simulink model "ObjectTrackerHDL_ew"  (R2024b)
settings: Solver=VariableStepAuto  StartTime=0.0  StopTime=0.2  RelTol=1e-3  EnableMultiTasking=on
PreLoadFcn:
  | % Blank input
  | img = zeros(480,640);
  | 
  | % Initialize ROI and its center
  | ROI = [175 270 127 127];
  | center = [ROI(2)+(ROI(4)+1)/2 ROI(1)+(ROI(3)+1)/2];
  | 
  | % Template Size
  | templateSize = 128;
  | tSize = templateSize;
  | 
  | % Learning rate
  | eta = 0.075;
  | 
  | % Number of training images
  | trainCount = 2;
  | 
  | % Gaussian Variance
  | sig = 2;
  | 
  | % Generate a Gaussian centered on the first frame
  | iSize = size(img);
  | [x,y] = ndgrid(1:iSize(1), 1:iSize(2));
  | gauss = exp(-((x-center(1)).^2 + (y-center(2)).^2)./(2*sig));
  | gauss = mat2gray(gauss);
  | 
  | % Generate the first template
  | img = imcrop(img, ROI);
  | gauss = imcrop(gauss, ROI);
  | 
  | % Generate the preprocess windowing function
  | [w1,w2] = meshgrid(window(@hann,tSize),window(@hann,tSize));
  | win = w1.*w2;
  | 
  | % Blank initial coefficients
  | G = zeros(tSize,tSize);
  | Ai = zeros(tSize,tSize);
  | Bi = zeros(tSize,tSize);
  | Hi = zeros(tSize,tSize);
  | 
  | numRows = tSize;
  | numCols = tSize;
InitFcn:
  | % Read the first frame
  | vidFReader = VideoReader(get_param('ObjectTrackerHDL/Input','inputFilename'));
  | img = read(vidFReader,1);
  | if (size(img,3) == 3)
  |     img = rgb2gray(img);
  | end
  | img = double(img);
  | 
  | % Initialize Object Center
  | objectCenter = str2num(get_param('ObjectTrackerHDL/ObjectTrackerHDL','objectCenter'));
  | 
  | % Template Size
  | templateSize = str2num(get_param('ObjectTrackerHDL/ObjectTrackerHDL','templateSize'));
  | originROI = objectCenter-templateSize/2;
  | tSize = templateSize;
  | 
  | % Initialize ROI and its center
  | ROI = [originROI tSize-1 tSize-1];
  | center = [ROI(2)+(ROI(4)+1)/2 ROI(1)+(ROI(3)+1)/2];
  | 
  | % Learning rate
  | eta = 0.075;
  | 
  | % Number of training images
  | trainCount = 128;
  | 
  | % Gaussian Variance
  | sig = 2;
  | 
  | % Generate a Gaussian centered on the first frame
  | iSize = size(img);
  | [x,y] = ndgrid(1:iSize(1), 1:iSize(2));
  | gauss = exp(-((x-center(1)).^2 + (y-center(2)).^2)./(2*sig));
  | gauss = mat2gray(gauss);
  | 
  | % Generate the first template
  | img = imcrop(img, ROI);
  | gauss = imcrop(gauss, ROI);
  | 
  | % Generate the preprocess windowing function
  | [w1,w2] = meshgrid(window(@hann,tSize),window(@hann,tSize));
  | win = w1.*w2;
  | 
  | % Preprocessing the first template
  | hgamma = vision.GammaCorrector(2.0,'Correction','De-gamma');
  | img = hgamma(uint8(img));
  | img = double(img);
  | mean1 = mean(img(:));
  | std1 = std(img(:));
  | img = (img-mean1)/std1;
  | fii = img.*win;
  | 
  | % Convert to frequency domain and calculate initial coefficients
  | G = fft2(gauss);
  | Ai = (G.*conj(fft2(fii)));
  | Bi = real((fft2(fii).*conj(fft2(fii))));
  | 
  | rng('default');
  | % Initial training procedure
  | for i = 1:trainCount
  |     rotateRand = 20.*rand - 10;
  |     resizeRand = 0.2.*rand + 0.9;
  |     img = imresize(imresize(imrotate(img, rotateRand), resizeRand), [tSize tSize]);
  |     img = hgamma(uint8(img));
  |     img = double(img);
  |     img = (img-mean(img(:)))/std(img(:));
  |     fii = img.*win;
  |     Ai = Ai + (G.*conj(fft2(fii)));
  |     Bi = Bi + real((fft2(fii).*conj(fft2(fii))));
  | end
  | 
  | % Initial Filter coefficients
  | Ai = eta.*Ai;
  | Bi = eta.*Bi;
  | Hi = Ai./Bi;
  | 
  | % FFT Parameters
  | numRows = tSize;
  | numCols = tSize;
model workspace (MAT data in the model file):
  mwTaskManagerKernelLatency = 0
undefined symbols (not defined in the file): a, b, c, Rec, SDTV
libraries: hdlsllib x61, simulink x17, visionhdlutilities x8, visionstatistics x6, dsphdlxfrm2 x6, visionconversions x4, visiontransforms x3, visionhdlio x2, visionhdlconversions x2, visionhdlstatistics x2, visionanalysis x2, visionsinks x1
(part 1 of 3)
settings Model: SimulationMode=accelerator  Creator=The MathWorks, Inc.  LastModifiedBy=samet
settings SolverCC: PositivePriorityOrder=on
settings OptimizationCC: BlockReduction=off  ConditionallyExecuteInputs=off  DefaultParameterBehavior=Inlined  EnhancedBackFolding=on  PassReuseOutputArgsAs=Individual arguments  ZeroExternalMemoryAtStartup=off  ZeroInternalMemoryAtStartup=off  MaxStackSize=64  OptimizeBlockOrder=speed  DifferentSizesBufferReuse=on  OptimizationCustomize=off  EfficientTunableParamExpr=on
settings DebuggingCC: AlgebraicLoopMsg=error  ParameterPrecisionLossMsg=none  ParameterTunabilityLossMsg=error  FixptConstOverflowMsg=warning  SubsystemReferenceDiagnosticForUnitTest=warning
settings HardwareCC: ProdBitPerPointer=32  ProdBitPerSizeT=32  ProdBitPerPtrDiffT=32  ProdLargestAtomicFloat=None  ProdIntDivRoundTo=Undefined  ProdEndianess=Unspecified  ProdWordSize=32  ProdHWDeviceType=ASIC/FPGA->ASIC/FPGA  TargetBitPerPointer=64  TargetBitPerSizeT=64  TargetBitPerPtrDiffT=64  TargetLongLongMode=on  TargetIntDivRoundTo=Zero  TargetEndianess=LittleEndian  TargetWordSize=64  TargetHWDeviceType=Custom Processor->MATLAB Host Computer  ProdEqTarget=off  HardwareBoardFeatureSet=SoCBlockset
settings ModelReferenceCC: ModelReferenceNumInstancesAllowed=Single
settings RTWCC: Description=Embedded Coder  SystemTargetFile=ert.tlc  TemplateMakefile=ert_default_tmf  Toolchain=Linaro AArch64 Linux v6.3.1  GPUComputeCapability=3.5
settings CodeAppCC: ForceParamTrailComments=on  IgnoreCustomStorageClasses=off  OperatorAnnotations=on  SimulinkDataObjDesc=on  SFDataObjDesc=on  InsertBlockDesc=on
settings ERTTargetCC: InlinedParameterPlacement=Hierarchical  ERTCustomFileTemplate=example_file_process.tlc  DynamicArrayContainerType=coder::array

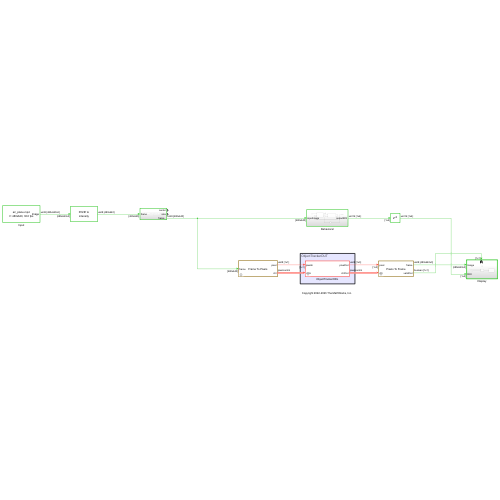
[thumbnail: Simulink's stored preview of the top-level diagram]
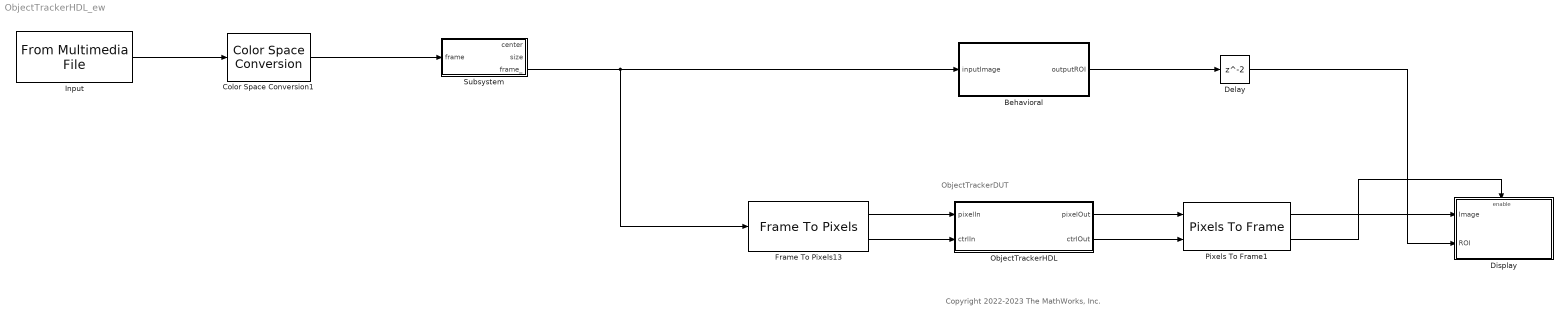
== system ObjectTrackerHDL_ew ==
  note: Copyright 2022-2023 The MathWorks, Inc.
  note: ObjectTrackerDUT
  Behavioral : Subsystem
  Color Space Conversion1 : visionconversions/Color Space  Conversion  conversion=Obsolete  conversionActive=R'G'B' to intensity  wp_str=D65  rec=Rec. 601 (SDTV)  sys=1125/60/2:1  imagePorts=One multidimensional signal
  Delay : Delay
  Display : Subsystem
  Frame To Pixels13 : visionhdlio/Frame To Pixels  NumComponents=1  NumPixels=1  VideoFormat=480p  ActivePixelsPerLine=640  ActiveVideoLines=480  TotalPixelsPerLine=800  TotalVideoLines=525  StartingActiveLine=36  FrontPorch=16  SampleTime=0  VideoFormatCache=480p  ActivePixelsPerLineCache=903  ActiveVideoLinesCache=718  TotalPixelsPerLineCache=950  TotalVideoLinesCache=750  StartingActiveLineCache=6  FrontPorchCache=5
  Input : dspvision/From Multimedia File  inputFilename=C:\Users\samet\OneDrive\Documents\MATLAB\Examples\R2024b\supportfiles\visionhdl\LTIR_dataset\air_plane.mp4  readRange=[1 Inf]  loop=on  numPlays=1  outputStreams=Video only  videoDataType=uint8  audioDataType=int16  inheritSampleTime=on  userDefinedSampleTime=1  noAudioOutput=off  isIntensityVideo=off  fourcc=RGB  colorVideoFormat=One multidimensional signal  outputEOF=off  dataOrg=Column-major  audioFrameSize=1024  computeAudioFrameSize=off  outSamplingMode=Sample based
      settings: LibrarySourceBlock=visionsources/From Multimedia File
  ObjectTrackerHDL : Subsystem  mask{objectCenter=[220 180], templateSize=128, imageSize=iSize}
      mask prompts: objectCenter "Object Center"; templateSize "Template Size"; imageSize "Image Size"
      mask init:
      | % Varsayılan edgeImage matrisi
      |     if evalin('base', 'exist(''edgeImage'', ''var'')') == 0
      |         defaultEdgeImage = false(480, 640); % Varsayılan boş edgeImage matrisi
      |         assignin('base', 'edgeImage', defaultEdgeImage);
      |         fprintf('edgeImage initialized to default zero matrix.\n');
      |     end
      | 
      |     % Retrieve edgeImage from the base workspace
      |     edgeImage = evalin('base', 'edgeImage');
      | 
      |     % Call calculateROI to compute objectCenter and templateSize
      |     try
      |         [objectCenter, templateSize] = calculateROI(edgeImage);
      |     catch ME
      |         error('Error in calculateROI: %s', ME.message);
      |     end
      | 
      |     % Assign computed values to the mask parameters
      |     assignin('base', 'objectCenter', objectCenter);
      |     assignin('base', 'templateSize', templateSize);
      | 
      |     % Debugging information
      |     fprintf('Initialization Complete:\n');
      |     fprintf('Object Center: [%f, %f]\n', objectCenter(1), objectCenter(2));
      |     fprintf('Template Size: %d\n', templateSize);
      mask TypeOptions templateSize: 16 | 32 | 64 | 128 | 256
  Pixels To Frame1 : visionhdlio/Pixels To Frame  NumComponents=3  NumPixels=1  VideoFormat=480p  ActivePixelsPerLine=640  ActiveVideoLines=480  TotalPixelsPerLine=800  TotalVideoLines=525  VideoFormatCache=480p  ActivePixelsPerLineCache=903  ActiveVideoLinesCache=718  TotalPixelsPerLineCache=950  TotalVideoLinesCache=750
  Subsystem : Subsystem
  wires:
  Frame To Pixels13/1 -> ObjectTrackerHDL/1(pixelIn)
  ObjectTrackerHDL/1(pixelOut) -> Pixels To Frame1/1
  ObjectTrackerHDL/2(ctrlOut) -> Pixels To Frame1/2
  Pixels To Frame1/2 -> Display/Enable
  Behavioral/1(outputROI) -> Delay/1
  Delay/1 -> Display/2(ROI)
  Input/1 -> Color Space Conversion1/1
  Frame To Pixels13/2 -> ObjectTrackerHDL/2(ctrlIn)
  Pixels To Frame1/1 -> Display/1(Image)
  Color Space Conversion1/1 -> Subsystem/1(frame)
  Subsystem/3(frame_) -> Frame To Pixels13/1, Behavioral/1(inputImage)

== system ObjectTrackerHDL_ew/Behavioral ==
  inputImage : Inport
  Preprocess : Subsystem
  Terminator : Terminator
  Track : Subsystem
  Transpose : Math  Operator=transpose
  outputROI : Outport
  wires:
  Preprocess/1(outputTemplate) -> Terminator/1
  Transpose/1 -> outputROI/1
  Preprocess/4(outputROI) -> Transpose/1
  inputImage/1 -> Preprocess/1(inputImage)
  Preprocess/2(prevTemplate) -> Track/1(prevTemplate)
  Preprocess/3(currTemplate) -> Track/2(currTemplate)
  Track/1(prevROI) -> Preprocess/2(prevROI)
  Track/2(currROI) -> Preprocess/3(currROI)

== system ObjectTrackerHDL_ew/Display ==
  Image : Inport
  ROI : Inport  Port=2
  Enable : EnablePort
  Display : visionsinks/To Video Display  windowSizeMode=Normal  openAtMdlStart=on  fullScreen=off  videoWindowX=536805376  videoWindowY=536805376  saveWindowSize=off  videoWindowWidth=1654  videoWindowHeight=1181  inputColorFormat=RGB  inputType=Obsolete  imagePorts=One multidimensional signal  OutputDevice=On-screen video monitor  dataOrg=Column-major  isWindowOpen=off
  VideoOverlay : MATLAB Function  TreatAsAtomicUnit=on
  wires:
  Image/1 -> VideoOverlay/1(img)
  VideoOverlay/1(y) -> Display/1
  ROI/1 -> VideoOverlay/2(ROI)

== system ObjectTrackerHDL_ew/ObjectTrackerHDL ==
  note: 2-D Correlation filter tracking HDL Subsystem
  pixelIn : Inport
  ctrlIn : Inport  Port=2
  Overlay : Subsystem
      settings: PortSchema="{\"entries\":[{\"content\":{\"sides\":[{\"content\":{\"connectorIds\":[\"In1\",\"In2\"]},\"type\":\"ConnectorPlacement.EquallySpacedRectSide\",\"uuid\":\"4b8534fb-eb59-4390-9dd3-f879eee42828\"},{\"content\":{\"connectorIds\":[\"Out1\",\"Out2\",\"Out3\"],\"side\":\"RIGHT\"},\"type\":\"ConnectorPlacement.EquallySpacedRectSide\",\"uuid\":\"fb136db1-f133-4b6e-b626-4dade9ce09b9\"},{\"content\":{\"connectorIds\":[\"In3\"],\"side\":\"TOP\"},\"type\":\"ConnectorPlacement.EquallySpacedRectSide\",\"uuid\":\"99d2356e-62e6-4658-9ddf-d950fdf75b9a\"}]},\"type\":\"ConnectorPlacement.EquallySpacedConnector\",\"uuid\":\"47760993-437f-4ecc-9b42-136ef2d923e2\"}],\"packageUris\":[\"http://schema.mathworks.com/mf0/Connector/R2020b\"],\"version\":\"1.0\"}"
  Preprocess : Subsystem
      settings: PortSchema="{\"entries\":[{\"content\":{\"sides\":[{\"content\":{\"connectorIds\":[\"In1\",\"In2\",\"In3\",\"In4\"]},\"type\":\"ConnectorPlacement.EquallySpacedRectSide\",\"uuid\":\"9cec2fe1-69b9-4dab-94c8-faa7de2288f4\"},{\"content\":{\"connectorIds\":[\"Out1\",\"Out2\",\"Out3\",\"Out4\"],\"side\":\"RIGHT\"},\"type\":\"ConnectorPlacement.EquallySpacedRectSide\",\"uuid\":\"e3a596ea-31b4-4396-a8e6-8b94a53ae325\"},{\"content\":{\"connectorIds\":[\"Out5\"],\"side\":\"TOP\"},\"type\":\"ConnectorPlacement.EquallySpacedRectSide\",\"uuid\":\"e24a773b-b8a7-44fa-b0cf-f932f975dd7c\"},{\"content\":{\"side\":\"BOTTOM\"},\"type\":\"ConnectorPlacement.EquallySpacedRectSide\",\"uuid\":\"5ab59a8a-723b-4ab7-825a-3368d576d645\"}]},\"type\":\"ConnectorPlacement.EquallySpacedConnector\",\"uuid\":\"d74f8764-7932-4caf-a531-fe5bd7d99976\"}],\"packageUris\":[\"http://schema.mathworks.com/mf0/Connector/R2020b\"],\"version\":\"1.0\"}"
  Terminator : Terminator
  Track : Subsystem
      settings: PortSchema="{\"entries\":[{\"content\":{\"sides\":[{\"content\":{\"connectorIds\":[\"In1\",\"In2\",\"In3\",\"In4\"]},\"type\":\"ConnectorPlacement.EquallySpacedRectSide\",\"uuid\":\"1d66b792-d543-473d-8440-e34f5801daf7\"},{\"content\":{\"connectorIds\":[\"Out1\",\"Out2\",\"In5\"],\"side\":\"RIGHT\"},\"type\":\"ConnectorPlacement.EquallySpacedRectSide\",\"uuid\":\"0e22f8bb-e063-4450-b36d-cf632a4b5b95\"},{\"content\":{\"side\":\"TOP\"},\"type\":\"ConnectorPlacement.EquallySpacedRectSide\",\"uuid\":\"c0411b5e-6970-47cf-84b0-714a2a15381e\"},{\"content\":{\"side\":\"BOTTOM\"},\"type\":\"ConnectorPlacement.EquallySpacedRectSide\",\"uuid\":\"e852d354-5e9d-40fe-bda7-81286cac12c5\"}]},\"type\":\"ConnectorPlacement.EquallySpacedConnector\",\"uuid\":\"8d3eada4-8f0a-418d-a426-b3492f84d556\"}],\"packageUris\":[\"http://schema.mathworks.com/mf0/Connector/R2020b\"],\"version\":\"1.0\"}"
  pixelOut : Outport
  ctrlOut : Outport  Port=2
  wires:
  ctrlIn/1 -> Overlay/2(ctrlIn), Track/5(frameCtrl), Preprocess/2(ctrlIn)
  pixelIn/1 -> Overlay/1(pixelIn), Preprocess/1(pixelIn)
  Preprocess/1(prevPixelOut) -> Track/1(prevPixelIn)
  Preprocess/2(prevCtrlOut) -> Track/2(prevCtrlIn)
  Preprocess/3(currPixelOut) -> Track/3(currPixelIn)
  Preprocess/4(currCtrlOut) -> Track/4(currCtrlIn)
  Track/1(prevROIOut) -> Preprocess/3(prevROI)
  Track/2(currROIOut) -> Preprocess/4(currROI)
  Preprocess/5(OutputROI) -> Overlay/3(ROIIn)
  Overlay/1(ROIOut) -> Terminator/1
  Overlay/2(pixelOut) -> pixelOut/1
  Overlay/3(ctrlOut) -> ctrlOut/1

== system ObjectTrackerHDL_ew/Subsystem ==
  frame : Inport
  Edge Detection : visionanalysis/Edge Detection  method=Prewitt  outputType=Binary image  userDefinedThreshold=off  thresholdSource=Input port  threshold=20  thresholdTuning=4  edgeThinning=off  threshold_canny=[0.25 0.60]  autoPercent=20  sigma=1  roundingMode=Floor  overflowMode=off  prodOutputMode=Binary point scaling  prodOutputWordLength=32  prodOutputFracLength=8
  Image Data Type Conversion1 : visionconversions/Image Data Type Conversion  outDT=uint8  isSigned=on  wordLen=16  numFracBits=0
  MATLAB Function : MATLAB Function  TreatAsAtomicUnit=on
  MATLAB Function1 : MATLAB Function
  Median Filter : visionanalysis/Median Filter  nghbood=[5 5]  outSize=Same as input port I  padType=Constant  padSrc=Specify via dialog  padVal=0  roundingMode=Floor  overflowMode=off
  Reshape : Reshape  OutputDimensionality=Row vector (2-D)  OutputDimensions=[1,2]
  Saturation : Saturate  UpperLimit=256  LowerLimit=16
  To Workspace : ToWorkspace  VariableName=edgeImage  SampleTime=-1
      settings: Save2DSignal=2-D array (concatenate along first dimension)
  center : Outport
  size : Outport  Port=2
  frame_ : Outport  Port=3
  wires:
  MATLAB Function1/2(templateSize) -> Saturation/1  "size"
  Reshape/1 -> center/1  "center"
  MATLAB Function1/1(objectCenter) -> Reshape/1
  Median Filter/1 -> MATLAB Function1/1("edgeImage ")
  Saturation/1 -> size/1
  MATLAB Function/1(outputImage) -> Edge Detection/1
  Image Data Type Conversion1/1 -> MATLAB Function/1(inputImage)
  frame/1 -> frame_/1, Image Data Type Conversion1/1
  Edge Detection/1 -> To Workspace/1, Median Filter/1

== system ObjectTrackerHDL_ew/Behavioral/Preprocess ==
  inputImage : Inport
  prevROI : Inport  Port=2
  currROI : Inport  Port=3
  Constant8 : Constant  Value=fi(win,0,16,16)  VectorParams1D=off  OutDataTypeStr=fixdt(0,16,16)  SampleTime=-1
  CurrPreprocess : Subsystem
  MATLAB Function1 : MATLAB Function  TreatAsAtomicUnit=on  mask{templateSize=tSize}
      mask prompts: templateSize "Template Size"
  MATLAB Function7 : MATLAB Function  TreatAsAtomicUnit=on  mask{templateSize=tSize}
      mask prompts: templateSize "Template Size"
  PrevPreprocess : Subsystem
  outputTemplate : Outport
  prevTemplate : Outport  Port=2
  currTemplate : Outport  Port=3
  outputROI : Outport  Port=4
  wires:
  MATLAB Function7/1(fi) -> outputTemplate/1, PrevPreprocess/1(in)
  CurrPreprocess/1(out) -> currTemplate/1
  Constant8/1 -> CurrPreprocess/2(window), PrevPreprocess/2(window)
  MATLAB Function1/1(fi) -> CurrPreprocess/1(in)
  PrevPreprocess/1(out) -> prevTemplate/1
  prevROI/1 -> outputROI/1, MATLAB Function7/2(ROI)
  inputImage/1 -> MATLAB Function1/1(img), MATLAB Function7/1(img)
  currROI/1 -> MATLAB Function1/2(ROI)

== system ObjectTrackerHDL_ew/Behavioral/Track ==
  prevTemplate : Inport
  currTemplate : Inport  Port=2
  2-DCorrelation : Subsystem
  MaxCorrelation : Subsystem
  ROIUpdate : Subsystem
  prevROI : Outport
  currROI : Outport  Port=2
  wires:
  currTemplate/1 -> 2-DCorrelation/2(currTemplate)
  ROIUpdate/2(currROI) -> currROI/1
  ROIUpdate/1(prevROI) -> prevROI/1
  prevTemplate/1 -> 2-DCorrelation/1(prevTemplate)
  MaxCorrelation/1(maxCol) -> ROIUpdate/1(maxCol)
  MaxCorrelation/2(maxRow) -> ROIUpdate/2(maxRow)
  2-DCorrelation/1(correlationOut) -> MaxCorrelation/1(correlationIn)

== system ObjectTrackerHDL_ew/ObjectTrackerHDL/Overlay ==
  note: Overlay Subsystem overlays the template bounding box onto the image frame
  pixelIn : Inport
  ctrlIn : Inport  Port=2
  ROIIn : Inport  Port=3
  Constant : Constant  OutDataTypeStr=uint16  SampleTime=-1
  Demux : Demux
  Mux : Mux
  Subtract : Sum  Inputs=+-  OutDataTypeStr=uint16
  Terminator2 : Terminator
  Vector Concatenate : Concatenate  NumInputs=4  Mode=Multidimensional array  ConcatenateDimension=2
  VideoOverlay : Subsystem  mask{color=Blue, opacity=1, mulChannel=off, numChannel=1, planeOpacity=0}
      mask prompts: opacity "Pixel Opacity"; mulChannel "Multiple Channels"; numChannel "Number of Channels"; planeOpacity "Plane Opacity"
      mask init:
      | %==========================================================================
      | % Get default values for optional parameters
      mask TypeOptions color: Red | Green | Blue | Cyan | Yellow
      mask TypeOptions numChannel: 1 | 2 | 3
      mask DialogControl Container2 Prompt: Multiple Channels
  ROIOut : Outport
  pixelOut : Outport  Port=2
  ctrlOut : Outport  Port=3
  wires:
  Demux/3 -> Subtract/1
  Constant/1 -> Subtract/2
  Demux/2 -> Vector Concatenate/1, Mux/2
  pixelIn/1 -> VideoOverlay/1(pixelIn)
  Vector Concatenate/1 -> VideoOverlay/3(Position)
  Subtract/1 -> Mux/4, Vector Concatenate/4, Vector Concatenate/3, Mux/3
  Demux/1 -> Mux/1, Vector Concatenate/2
  Demux/4 -> Terminator2/1
  VideoOverlay/2(ctrlOut) -> ctrlOut/1
  VideoOverlay/1(pixelOut) -> pixelOut/1
  ROIIn/1 -> Demux/1
  Mux/1 -> ROIOut/1
  ctrlIn/1 -> VideoOverlay/2(ctrlIn)

== system ObjectTrackerHDL_ew/ObjectTrackerHDL/Preprocess ==
  note: Preprocess Subsystem selects the templates and does mean subtraction, variance normalization and windowing
  pixelIn : Inport
  ctrlIn : Inport  Port=2
  prevROI : Inport  Port=3
  currROI : Inport  Port=4
  1-D Lookup Table : Lookup_n-D  NumberOfTableDimensions=1  LookupTableObject=''  BreakpointsForDimension1=[0:tSize * tSize - 1]  BreakpointsForDimension1FirstPoint=10  BreakpointsForDimension2FirstPoint=10  BreakpointsForDimension1Spacing=12  BreakpointsForDimension2Spacing=12  IndexSearchMethod=Evenly spaced points  Table=fi(win(:)',0,16,16)  InterpMethod=Flat  DiagnosticForOutOfRangeInput=Error  InternalRulePriority=Speed  OutDataTypeStr=fixdt(0,16,16)  RndMeth=Simplest
  Constant : Constant  Value=0  OutDataTypeStr=boolean  SampleTime=-1
  CurrPreprocess : Subsystem
  Delay : Delay  DelayLength=1
  HDL Counter : hdlsllib/Sources/HDL Counter  CountType=Count limited  CountInit=0  CountStep=1  CountMax=tSize * tSize - 1  CountFromType=Initial value  CountFrom=0  CountResetPort=on  CountLoadPort=off  CountEnbPort=on  CountDirPort=off  CountHitOutputPort=off  CountDataType=Unsigned  CountWordLen=ceil(log2(tSize * tSize - 1))  CountFracLen=0  CountSampTime=1
  Pixel Control Bus Selector : BusSelector  OutputSignals=valid
  PrevPreprocess : Subsystem
  ROI Selector : visionhdlutilities/ROI Selector  VerticalReuse=off  RegionsSource=Input port  NumberOfRegions=1  Regions=[100 100 50 50]  SimulateUsing=Code generation
  ROI Selector1 : visionhdlutilities/ROI Selector  VerticalReuse=off  RegionsSource=Input port  NumberOfRegions=1  Regions=[100 100 50 50]  SimulateUsing=Code generation
  prevPixelOut : Outport
  prevCtrlOut : Outport  Port=2
  currPixelOut : Outport  Port=3
  currCtrlOut : Outport  Port=4
  OutputROI : Outport  Port=5
  wires:
  currROI/1 -> ROI Selector1/3
  ROI Selector1/2 -> CurrPreprocess/3(ctrlIn)
  CurrPreprocess/2(ctrlOut) -> currCtrlOut/1
  Pixel Control Bus Selector/1 -> HDL Counter/2  "<valid>"
  1-D Lookup Table/1 -> Delay/1
  HDL Counter/1 -> 1-D Lookup Table/1
  ROI Selector/1 -> PrevPreprocess/1(pixelIn)
  Constant/1 -> HDL Counter/1
  ROI Selector1/1 -> CurrPreprocess/1(pixelIn)
  ROI Selector/2 -> Pixel Control Bus Selector/1, PrevPreprocess/3(ctrlIn)
  PrevPreprocess/1(pixelOut) -> prevPixelOut/1
  CurrPreprocess/1(pixelOut) -> currPixelOut/1
  prevROI/1 -> OutputROI/1, ROI Selector/3
  PrevPreprocess/2(ctrlOut) -> prevCtrlOut/1
  pixelIn/1 -> ROI Selector1/1, ROI Selector/1
  ctrlIn/1 -> PrevPreprocess/4(frameCtrl), CurrPreprocess/4(frameCtrl), ROI Selector1/2, ROI Selector/2
  Delay/1 -> PrevPreprocess/2(pixelWindow), CurrPreprocess/2(pixelWindow)

== system ObjectTrackerHDL_ew/ObjectTrackerHDL/Track ==
  note: Tracking HDL Subsystem performs 2D correlation, calculates maximum of 2D correlation point and updates the ROI
  prevPixelIn : Inport
  prevCtrlIn : Inport  Port=2
  currPixelIn : Inport  Port=3
  currCtrlIn : Inport  Port=4
  frameCtrl : Inport  Port=5
  2-DCorrelation : Subsystem
      settings: PortSchema="{\"entries\":[{\"content\":{\"sides\":[{\"content\":{\"connectorIds\":[\"In1\",\"In2\",\"In3\",\"In4\",\"In5\"]},\"type\":\"ConnectorPlacement.EquallySpacedRectSide\",\"uuid\":\"7528fa5d-0ab3-4341-8e98-b9271544417e\"},{\"content\":{\"connectorIds\":[\"Out1\",\"Out2\"],\"side\":\"RIGHT\"},\"type\":\"ConnectorPlacement.EquallySpacedRectSide\",\"uuid\":\"72d4aff4-65e1-4e65-bf4f-ba7a8870cbfa\"},{\"content\":{\"connectorIds\":[\"In6\"],\"side\":\"TOP\"},\"type\":\"ConnectorPlacement.EquallySpacedRectSide\",\"uuid\":\"4516de4b-a47c-40bd-acbe-eaa29e8d8289\"}]},\"type\":\"ConnectorPlacement.EquallySpacedConnector\",\"uuid\":\"f94c40d7-16f2-4e10-b02c-2b09c4adb3bf\"}],\"packageUris\":[\"http://schema.mathworks.com/mf0/Connector/R2020b\"],\"version\":\"1.0\"}"
  Delay7 : Delay  DelayLength=20
  MaxCorrelation : Subsystem
  ROIUpdate : Subsystem
  prevROIOut : Outport
  currROIOut : Outport  Port=2
  wires:
  ROIUpdate/2(prevROI) -> prevROIOut/1
  2-DCorrelation/1(pixelOut) -> MaxCorrelation/1(pixelIn)
  prevPixelIn/1 -> 2-DCorrelation/1(prevPixelIn)
  currCtrlIn/1 -> 2-DCorrelation/4(currCtrlIn)
  2-DCorrelation/2(ctrlOut) -> MaxCorrelation/2(ctrlIn)
  currPixelIn/1 -> 2-DCorrelation/3(currPixelIn)
  ROIUpdate/1(streamCtrlOut) -> 2-DCorrelation/5(streamCtrlIn)
  prevCtrlIn/1 -> 2-DCorrelation/2(prevCtrlIn)
  ROIUpdate/3(currROI) -> currROIOut/1
  frameCtrl/1 -> MaxCorrelation/3(frameCtrl), 2-DCorrelation/6(frameCtrl), Delay7/1
  MaxCorrelation/1(maxCol) -> ROIUpdate/1(maxCol)
  MaxCorrelation/2(maxRow) -> ROIUpdate/2(maxRow)
  Delay7/1 -> ROIUpdate/3(frameCtrl)

== system ObjectTrackerHDL_ew/Behavioral/Preprocess/CurrPreprocess ==
  in : Inport
  window : Inport  Port=2
  2-D Mean2 : visionstatistics/2-D Mean  run=off  reset_popup=None  directionMode=Entire input  dimension=1  treatSBRowAsCol=on  outputMode=Binary point scaling  outputWordLength=8  outputFracLength=0  outputLastDataTypeStr=fixdt([],8,0)  accumMode=Binary point scaling  accumWordLength=32  accumFracLength=0  accumLastDataTypeStr=fixdt([],32,0)  roiEnable=off  roiType=Rectangles  roiPortion=Entire ROI  roiOutput=Individual statistics for each ROI  roiFlag=off  roundingMode=Floor  overflowMode=on  accumDataTypeStr=fixdt([],32,0)  outputDataTypeStr=fixdt([],8,0)  outputMin=[]  outputMax=[]
  2-D Standard Deviation : visionstatistics/2-D Standard Deviation  run=off  reset_popup=None  InputProcessing=Columns as channels (frame based)  directionMode=Entire input  dimension=1  treatSBRowAsCol=on  roiEnable=off  roiType=Rectangles  roiPortion=Entire ROI  roiOutput=Individual statistics for each ROI  roiFlag=off
  Data Type Conversion2 : DataTypeConversion  OutDataTypeStr=uint8  SaturateOnIntegerOverflow=off  RndMeth=Floor
  Data Type Conversion3 : DataTypeConversion  OutDataTypeStr=single  SaturateOnIntegerOverflow=off  RndMeth=Floor
  Delay : Delay  DelayLength=1  InitialCondition=uint8(mean1)
  Delay1 : Delay  DelayLength=1  InitialCondition=uint8(std1)
  Divide1 : Product  Inputs=*/  OutDataTypeStr=fixdt(1,16,12)  SaturateOnIntegerOverflow=on
  Gamma Correction : visionconversions/Gamma Correction  operation=De-gamma  gamma=2  linearSegment=on  breakPoint=0.018
  Product : Product
  Subtract2 : Sum  Inputs=+-  OutDataTypeStr=fixdt(1,16,0)
  out : Outport
  wires:
  Gamma Correction/1 -> Data Type Conversion3/1, 2-D Mean2/1, Subtract2/1
  2-D Standard Deviation/1 -> Data Type Conversion2/1
  Data Type Conversion2/1 -> Delay1/1
  in/1 -> Gamma Correction/1
  Divide1/1 -> Product/1
  2-D Mean2/1 -> Delay/1
  Data Type Conversion3/1 -> 2-D Standard Deviation/1
  Subtract2/1 -> Divide1/1
  window/1 -> Product/2
  Product/1 -> out/1
  Delay1/1 -> Divide1/2
  Delay/1 -> Subtract2/2

== system ObjectTrackerHDL_ew/Behavioral/Preprocess/PrevPreprocess ==
  in : Inport
  window : Inport  Port=2
  2-D Mean2 : visionstatistics/2-D Mean  run=off  reset_popup=None  directionMode=Entire input  dimension=1  treatSBRowAsCol=on  outputMode=Binary point scaling  outputWordLength=8  outputFracLength=0  outputLastDataTypeStr=fixdt([],8,0)  accumMode=Binary point scaling  accumWordLength=32  accumFracLength=0  accumLastDataTypeStr=fixdt([],32,0)  roiEnable=off  roiType=Rectangles  roiPortion=Entire ROI  roiOutput=Individual statistics for each ROI  roiFlag=off  roundingMode=Floor  overflowMode=on  accumDataTypeStr=fixdt([],32,0)  outputDataTypeStr=fixdt([],8,0)  outputMin=[]  outputMax=[]
  2-D Standard Deviation : visionstatistics/2-D Standard Deviation  run=off  reset_popup=None  InputProcessing=Columns as channels (frame based)  directionMode=Entire input  dimension=1  treatSBRowAsCol=on  roiEnable=off  roiType=Rectangles  roiPortion=Entire ROI  roiOutput=Individual statistics for each ROI  roiFlag=off
  Data Type Conversion2 : DataTypeConversion  OutDataTypeStr=uint8  SaturateOnIntegerOverflow=off  RndMeth=Floor
  Data Type Conversion3 : DataTypeConversion  OutDataTypeStr=single  SaturateOnIntegerOverflow=off  RndMeth=Floor
  Delay : Delay  DelayLength=1  InitialCondition=uint8(mean1)
  Delay1 : Delay  DelayLength=1  InitialCondition=uint8(std1)
  Divide1 : Product  Inputs=*/  OutDataTypeStr=fixdt(1,16,12)  SaturateOnIntegerOverflow=on
  Gamma Correction : visionconversions/Gamma Correction  operation=De-gamma  gamma=2  linearSegment=on  breakPoint=0.018
  Product : Product
  Subtract2 : Sum  Inputs=+-  OutDataTypeStr=fixdt(1,16,0)
  out : Outport
  wires:
  Gamma Correction/1 -> Data Type Conversion3/1, 2-D Mean2/1, Subtract2/1
  2-D Standard Deviation/1 -> Data Type Conversion2/1
  Data Type Conversion2/1 -> Delay1/1
  in/1 -> Gamma Correction/1
  Divide1/1 -> Product/1
  2-D Mean2/1 -> Delay/1
  Data Type Conversion3/1 -> 2-D Standard Deviation/1
  Subtract2/1 -> Divide1/1
  window/1 -> Product/2
  Product/1 -> out/1
  Delay/1 -> Subtract2/2
  Delay1/1 -> Divide1/2

== system ObjectTrackerHDL_ew/Behavioral/Track/2-DCorrelation ==
  prevTemplate : Inport
  currTemplate : Inport  Port=2
  2-D FFT : visiontransforms/2-D FFT  TableOpt=NEW  TableOptActive=Speed  FFTImplementation=Auto  BitRevOrder=off  SkipNorm=off  firstCoeffLastDataTypeStr=Inherit: Same word length as input  outputMode=Binary point scaling  outputWordLength=24  outputFracLength=12  outputLastDataTypeStr=fixdt(1,24,12)  roundingMode=Floor  overflowMode=off  firstCoeffDataTypeStr=Inherit: Same word length as input  outputDataTypeStr=fixdt(1,24,12)  outputMin=[]  outputMax=[]
  2-D FFT1 : visiontransforms/2-D FFT  TableOpt=NEW  TableOptActive=Speed  FFTImplementation=Auto  BitRevOrder=off  SkipNorm=off  firstCoeffLastDataTypeStr=Inherit: Same word length as input  outputMode=Binary point scaling  outputWordLength=24  outputFracLength=12  outputLastDataTypeStr=fixdt(1,24,12)  roundingMode=Floor  overflowMode=off  firstCoeffDataTypeStr=Inherit: Same word length as input  outputDataTypeStr=fixdt(1,24,12)  outputMin=[]  outputMax=[]
  2-D IFFT : visiontransforms/2-D IFFT  TableOpt=NEW  TableOptActive=Speed  FFTImplementation=Auto  BitRevOrder=off  cs_in=off  divideOutput=on  SkipNorm=on  firstCoeffLastDataTypeStr=Inherit: Same word length as input  outputMode=Binary point scaling  outputWordLength=24  outputFracLength=16  outputLastDataTypeStr=fixdt(1,24,16)  roundingMode=Floor  overflowMode=off  firstCoeffDataTypeStr=Inherit: Same word length as input  outputDataTypeStr=fixdt(1,24,16)  outputMin=[]  outputMax=[]
  CoefficientsUpdate : Subsystem
  Product8 : Product  OutDataTypeStr=fixdt(1,24,16)
  Transpose : Math  Operator=transpose
  Transpose1 : Math  Operator=transpose
  Transpose2 : Math  Operator=transpose
  correlationOut : Outport
  wires:
  prevTemplate/1 -> 2-D FFT/1
  CoefficientsUpdate/1(Out) -> Product8/2
  2-D FFT/1 -> Transpose/1
  Product8/1 -> 2-D IFFT/1
  2-D IFFT/1 -> Transpose2/1
  Transpose/1 -> Product8/1
  currTemplate/1 -> 2-D FFT1/1
  2-D FFT1/1 -> Transpose1/1
  Transpose1/1 -> CoefficientsUpdate/1(In)
  Transpose2/1 -> correlationOut/1

== system ObjectTrackerHDL_ew/Behavioral/Track/MaxCorrelation ==
  correlationIn : Inport
  2-D Mean3 : visionstatistics/2-D Mean  run=off  reset_popup=None  directionMode=Entire input  dimension=1  treatSBRowAsCol=on  outputLastDataTypeStr=Inherit: Same as accumulator  accumMode=Binary point scaling  accumWordLength=16  accumFracLength=0  accumLastDataTypeStr=fixdt([],16,0)  roiEnable=off  roiType=Rectangles  roiPortion=Entire ROI  roiOutput=Individual statistics for each ROI  roiFlag=off  roundingMode=Floor  overflowMode=off  accumDataTypeStr=fixdt([],16,0)  outputDataTypeStr=Inherit: Same as accumulator  outputMin=[]  outputMax=[]
  2-D Mean4 : visionstatistics/2-D Mean  run=off  reset_popup=None  directionMode=Entire input  dimension=1  treatSBRowAsCol=on  outputLastDataTypeStr=Inherit: Same as accumulator  accumMode=Binary point scaling  accumWordLength=16  accumFracLength=0  accumLastDataTypeStr=fixdt([],16,0)  roiEnable=off  roiType=Rectangles  roiPortion=Entire ROI  roiOutput=Individual statistics for each ROI  roiFlag=off  roundingMode=Floor  overflowMode=off  accumDataTypeStr=fixdt([],16,0)  outputDataTypeStr=Inherit: Same as accumulator  outputMin=[]  outputMax=[]
  Complex to Real-Imag : ComplexToRealImag
  Data Type Conversion1 : DataTypeConversion  OutDataTypeStr=uint16  SaturateOnIntegerOverflow=off  RndMeth=Floor
  Data Type Conversion3 : DataTypeConversion  OutDataTypeStr=single  SaturateOnIntegerOverflow=off  RndMeth=Floor
  Data Type Conversion4 : DataTypeConversion  OutDataTypeStr=uint16  SaturateOnIntegerOverflow=off  RndMeth=Floor
  MATLAB Function13 : MATLAB Function  TreatAsAtomicUnit=on
  Terminator : Terminator
  maxCol : Outport
  maxRow : Outport  Port=2
  wires:
  Complex to Real-Imag/1 -> MATLAB Function13/1(gi)
  Complex to Real-Imag/2 -> Terminator/1
  MATLAB Function13/2(Q) -> Data Type Conversion4/1
  Data Type Conversion4/1 -> 2-D Mean4/1
  Data Type Conversion1/1 -> 2-D Mean3/1
  Data Type Conversion3/1 -> Complex to Real-Imag/1
  2-D Mean3/1 -> maxCol/1
  MATLAB Function13/1(P) -> Data Type Conversion1/1
  2-D Mean4/1 -> maxRow/1
  correlationIn/1 -> Data Type Conversion3/1

== system ObjectTrackerHDL_ew/Behavioral/Track/ROIUpdate ==
  maxCol : Inport
  maxRow : Inport  Port=2
  Add4 : Sum  OutDataTypeStr=uint16
  Add5 : Sum  OutDataTypeStr=uint16
  CurrValidROI : Subsystem
  Delay7 : Delay  DelayLength=1  InitialConditionSource=Input port  InitialCondition=0
      settings: InputPortMap=u0,p4
  Demux1 : Demux
  Mux1 : Mux
  PrevValidROI : Subsystem
  ROI : Constant  Value=uint16(ROI)  OutDataTypeStr=uint16  SampleTime=-1
  Subtract3 : Sum  Inputs=+-  OutDataTypeStr=fixdt(1,17,0)
  Subtract4 : Sum  Inputs=+-  OutDataTypeStr=fixdt(1,17,0)
  height/2 : Constant  Value=uint16(tSize/2)  SampleTime=-1
  width/2 : Constant  Value=uint16(tSize/2)  SampleTime=-1
  prevROI : Outport
  currROI : Outport  Port=2
  wires:
  maxCol/1 -> Subtract3/1
  height/2/1 -> Subtract3/2
  Demux1/2 -> Add4/2
  Demux1/3 -> Mux1/3
  Demux1/4 -> Mux1/4
  Subtract4/1 -> Add5/1
  width/2/1 -> Subtract4/2
  Add4/1 -> Mux1/2
  Add5/1 -> Mux1/1
  Subtract3/1 -> Add4/1
  Demux1/1 -> Add5/2
  maxRow/1 -> Subtract4/1
  PrevValidROI/1(ROIOut) -> prevROI/1
  CurrValidROI/1(ROIOut) -> currROI/1
  ROI/1 -> Delay7/2
  Delay7/1 -> PrevValidROI/1(ROIIn), Demux1/1
  Mux1/1 -> Delay7/1, CurrValidROI/1(ROIIn)

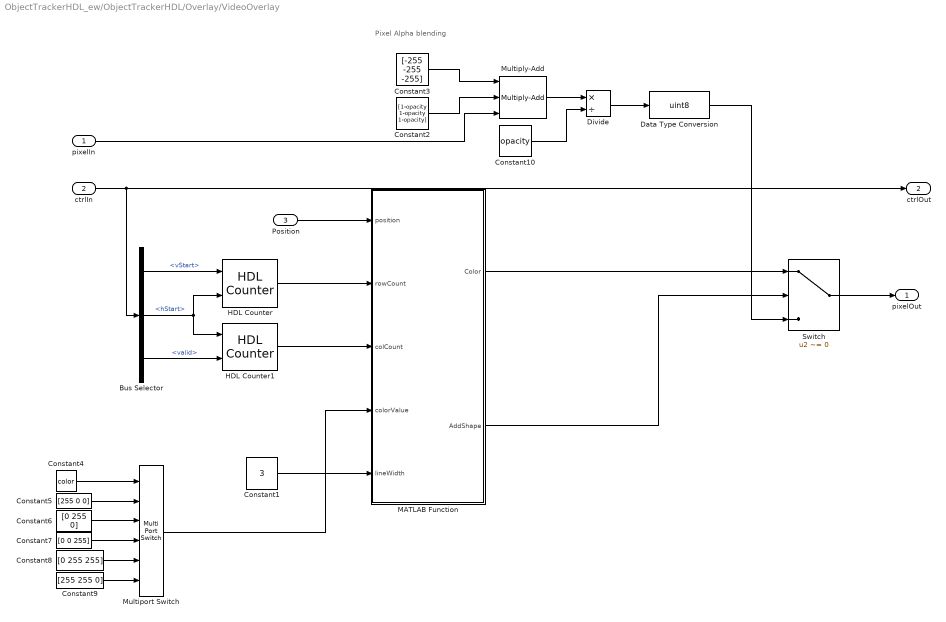
== system ObjectTrackerHDL_ew/ObjectTrackerHDL/Overlay/VideoOverlay ==
  note: Pixel Alpha blending
  pixelIn : Inport
  ctrlIn : Inport  Port=2
  Position : Inport  Port=3
  Bus Selector : BusSelector  OutputSignals=vStart,hStart,valid
  Constant1 : Constant  Value=3  VectorParams1D=off  OutDataTypeStr=uint8  SampleTime=-1
  Constant10 : Constant  Value=opacity  VectorParams1D=off  OutDataTypeStr=int8  SampleTime=-1
  Constant2 : Constant  Value=[1-opacity 1-opacity 1-opacity]  VectorParams1D=off  OutDataTypeStr=int8  SampleTime=-1
  Constant3 : Constant  Value=[-255 -255 -255]  VectorParams1D=off  OutDataTypeStr=fixdt(1,9,0)  SampleTime=-1
  Constant4 : Constant  Value=color  OutDataTypeStr=uint8  SampleTime=-1
  Constant5 : Constant  Value=[255 0 0]  VectorParams1D=off  OutDataTypeStr=uint8  SampleTime=-1
  Constant6 : Constant  Value=[0 255 0]  VectorParams1D=off  OutDataTypeStr=uint8  SampleTime=-1
  Constant7 : Constant  Value=[0 0 255]  VectorParams1D=off  OutDataTypeStr=uint8  SampleTime=-1
  Constant8 : Constant  Value=[0 255 255]  VectorParams1D=off  OutDataTypeStr=uint8  SampleTime=-1
  Constant9 : Constant  Value=[255 255 0]  VectorParams1D=off  OutDataTypeStr=uint8  SampleTime=-1
  Data Type Conversion : DataTypeConversion  OutDataTypeStr=uint8  SaturateOnIntegerOverflow=off  RndMeth=Floor
  Divide : Product  Inputs=*/  RndMeth=Zero  SaturateOnIntegerOverflow=on
  HDL Counter : hdlsllib/Sources/HDL Counter  CountType=Free running  CountInit=0  CountStep=1  CountMax=240  CountFromType=Initial value  CountFrom=0  CountResetPort=on  CountLoadPort=off  CountEnbPort=on  CountDirPort=off  CountHitOutputPort=off  CountDataType=Signed  CountWordLen=32  CountFracLen=0  CountSampTime=1
  HDL Counter1 : hdlsllib/Sources/HDL Counter  CountType=Free running  CountInit=0  CountStep=1  CountMax=360  CountFromType=Initial value  CountFrom=0  CountResetPort=on  CountLoadPort=off  CountEnbPort=on  CountDirPort=off  CountHitOutputPort=off  CountDataType=Signed  CountWordLen=32  CountFracLen=0  CountSampTime=1
  MATLAB Function : MATLAB Function  TreatAsAtomicUnit=on
  Multiply-Add : hdlsllib/HDL Operations/Multiply-Add  Function=c+(a.*b)  datatype=Inherit: Inherit via internal rule  DoSatur=off  FMA=off
  Multiport Switch : MultiPortSwitch  Inputs=5  SaturateOnIntegerOverflow=off  InputSameDT=off
  Switch : Switch  Criteria=u2 ~= 0  SaturateOnIntegerOverflow=off  InputSameDT=off
  pixelOut : Outport
  ctrlOut : Outport  Port=2
  wires:
  HDL Counter1/1 -> MATLAB Function/3(colCount)
  ctrlIn/1 -> Bus Selector/1, ctrlOut/1
  Position/1 -> MATLAB Function/1(position)
  HDL Counter/1 -> MATLAB Function/2(rowCount)
  MATLAB Function/2(AddShape) -> Switch/2
  MATLAB Function/1(Color) -> Switch/1
  pixelIn/1 -> Multiply-Add/3
  Switch/1 -> pixelOut/1
  Bus Selector/1 -> HDL Counter/1  "<vStart>"
  Bus Selector/3 -> HDL Counter1/2  "<valid>"
  Bus Selector/2 -> HDL Counter/2, HDL Counter1/1  "<hStart>"
  Multiport Switch/1 -> MATLAB Function/4(colorValue)
  Constant1/1 -> MATLAB Function/5(lineWidth)
  Constant2/1 -> Multiply-Add/2
  Constant3/1 -> Multiply-Add/1
  Multiply-Add/1 -> Divide/1
  Divide/1 -> Data Type Conversion/1
  Data Type Conversion/1 -> Switch/3
  Constant4/1 -> Multiport Switch/1
  Constant5/1 -> Multiport Switch/2
  Constant6/1 -> Multiport Switch/3
  Constant7/1 -> Multiport Switch/4
  Constant8/1 -> Multiport Switch/5
  Constant9/1 -> Multiport Switch/6
  Constant10/1 -> Divide/2

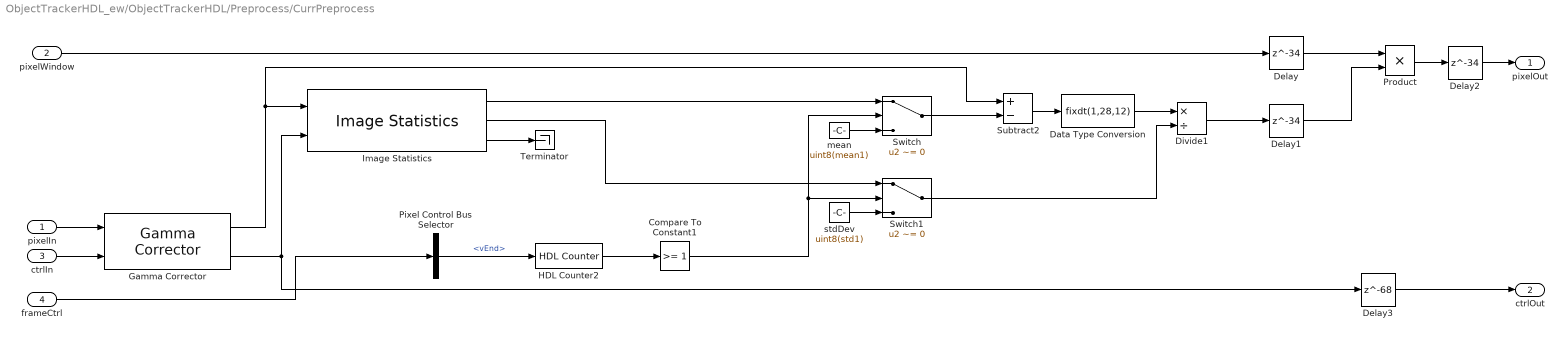
== system ObjectTrackerHDL_ew/ObjectTrackerHDL/Preprocess/CurrPreprocess ==
  pixelIn : Inport
  pixelWindow : Inport  Port=2
  ctrlIn : Inport  Port=3
  frameCtrl : Inport  Port=4
  Compare To Constant1 : simulink/Logic and Bit Operations/Compare To Constant  relop=>=  const=1  OutDataTypeStr=boolean
  Data Type Conversion : DataTypeConversion  OutDataTypeStr=fixdt(1,28,12)  SaturateOnIntegerOverflow=off  RndMeth=Floor
  Delay : Delay  DelayLength=34
  Delay1 : Delay  DelayLength=34
  Delay2 : Delay  DelayLength=34
  Delay3 : Delay  DelayLength=68
  Divide1 : Product  Inputs=*/  OutDataTypeStr=fixdt(1,16,12)  RndMeth=Zero  SaturateOnIntegerOverflow=on
  Gamma Corrector : visionhdlconversions/Gamma Corrector  Correction=De-gamma  Gamma=2  LinearSegment=on  BreakPoint=0.018  SimulateUsing=Code generation
  HDL Counter2 : hdlsllib/Sources/HDL Counter  CountType=Count limited  CountInit=0  CountStep=1  CountMax=4095  CountFromType=Initial value  CountFrom=0  CountResetPort=off  CountLoadPort=off  CountEnbPort=on  CountDirPort=off  CountHitOutputPort=off  CountDataType=Unsigned  CountWordLen=12  CountFracLen=0  CountSampTime=1
  Image Statistics : visionhdlstatistics/Image Statistics  mean=on  variance=off  stdDev=on  SimulateUsing=Code generation
  Pixel Control Bus Selector : BusSelector  OutputSignals=vEnd
  Product : Product
  Subtract2 : Sum  Inputs=+-  OutDataTypeStr=fixdt(1,16,0)
  Switch : Switch  Criteria=u2 ~= 0  SaturateOnIntegerOverflow=off  InputSameDT=off
  Switch1 : Switch  Criteria=u2 ~= 0  SaturateOnIntegerOverflow=off  InputSameDT=off
  Terminator : Terminator
  mean : Constant  Value=uint8(mean1)  OutDataTypeStr=uint8  SampleTime=-1
  stdDev : Constant  Value=uint8(std1)  OutDataTypeStr=uint8  SampleTime=-1
  pixelOut : Outport
  ctrlOut : Outport  Port=2
  wires:
  Subtract2/1 -> Data Type Conversion/1
  Gamma Corrector/1 -> Image Statistics/1, Subtract2/1
  Gamma Corrector/2 -> Delay3/1, Image Statistics/2
  pixelIn/1 -> Gamma Corrector/1
  ctrlIn/1 -> Gamma Corrector/2
  Product/1 -> Delay2/1
  Switch/1 -> Subtract2/2
  HDL Counter2/1 -> Compare To Constant1/1
  mean/1 -> Switch/3
  stdDev/1 -> Switch1/3
  Image Statistics/2 -> Switch1/1
  Image Statistics/1 -> Switch/1
  Pixel Control Bus Selector/1 -> HDL Counter2/1  "<vEnd>"
  Compare To Constant1/1 -> Switch1/2, Switch/2
  Divide1/1 -> Delay1/1
  pixelWindow/1 -> Delay/1
  Data Type Conversion/1 -> Divide1/1
  Switch1/1 -> Divide1/2
  Image Statistics/3 -> Terminator/1
  frameCtrl/1 -> Pixel Control Bus Selector/1
  Delay/1 -> Product/1
  Delay1/1 -> Product/2
  Delay2/1 -> pixelOut/1
  Delay3/1 -> ctrlOut/1

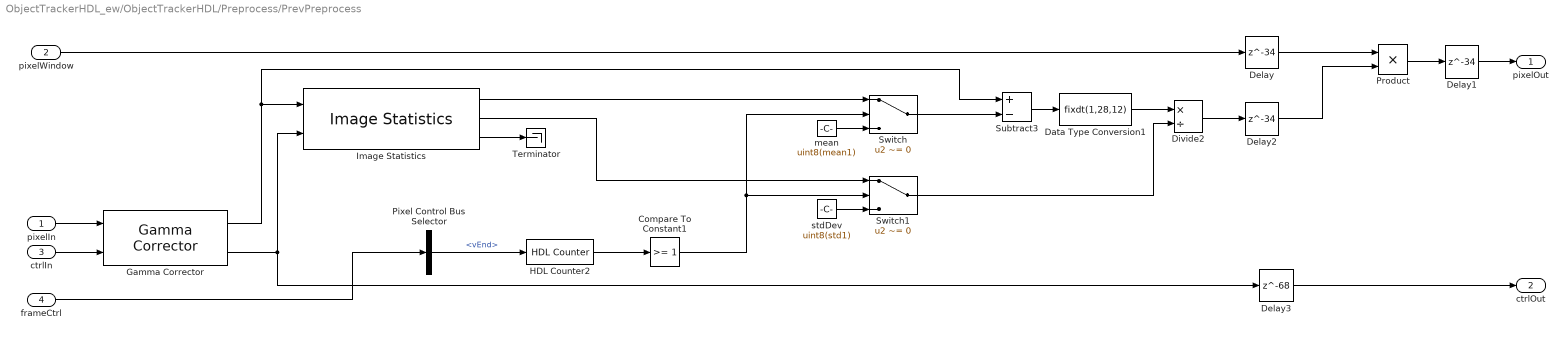
== system ObjectTrackerHDL_ew/ObjectTrackerHDL/Preprocess/PrevPreprocess ==
  pixelIn : Inport
  pixelWindow : Inport  Port=2
  ctrlIn : Inport  Port=3
  frameCtrl : Inport  Port=4
  Compare To Constant1 : simulink/Logic and Bit Operations/Compare To Constant  relop=>=  const=1  OutDataTypeStr=boolean
  Data Type Conversion1 : DataTypeConversion  OutDataTypeStr=fixdt(1,28,12)  SaturateOnIntegerOverflow=off  RndMeth=Floor
  Delay : Delay  DelayLength=34
  Delay1 : Delay  DelayLength=34
  Delay2 : Delay  DelayLength=34
  Delay3 : Delay  DelayLength=68
  Divide2 : Product  Inputs=*/  OutDataTypeStr=fixdt(1,16,12)  RndMeth=Zero  SaturateOnIntegerOverflow=on
  Gamma Corrector : visionhdlconversions/Gamma Corrector  Correction=De-gamma  Gamma=2  LinearSegment=on  BreakPoint=0.018  SimulateUsing=Code generation
  HDL Counter2 : hdlsllib/Sources/HDL Counter  CountType=Count limited  CountInit=0  CountStep=1  CountMax=4095  CountFromType=Initial value  CountFrom=0  CountResetPort=off  CountLoadPort=off  CountEnbPort=on  CountDirPort=off  CountHitOutputPort=off  CountDataType=Unsigned  CountWordLen=12  CountFracLen=0  CountSampTime=1
  Image Statistics : visionhdlstatistics/Image Statistics  mean=on  variance=off  stdDev=on  SimulateUsing=Code generation
  Pixel Control Bus Selector : BusSelector  OutputSignals=vEnd
  Product : Product
  Subtract3 : Sum  Inputs=+-  OutDataTypeStr=fixdt(1,16,0)
  Switch : Switch  Criteria=u2 ~= 0  SaturateOnIntegerOverflow=off  InputSameDT=off
  Switch1 : Switch  Criteria=u2 ~= 0  SaturateOnIntegerOverflow=off  InputSameDT=off
  Terminator : Terminator
  mean : Constant  Value=uint8(mean1)  OutDataTypeStr=uint8  SampleTime=-1
  stdDev : Constant  Value=uint8(std1)  OutDataTypeStr=uint8  SampleTime=-1
  pixelOut : Outport
  ctrlOut : Outport  Port=2
  wires:
  Gamma Corrector/1 -> Image Statistics/1, Subtract3/1
  Gamma Corrector/2 -> Delay3/1, Image Statistics/2
  pixelIn/1 -> Gamma Corrector/1
  ctrlIn/1 -> Gamma Corrector/2
  Product/1 -> Delay1/1
  HDL Counter2/1 -> Compare To Constant1/1
  mean/1 -> Switch/3
  stdDev/1 -> Switch1/3
  Image Statistics/2 -> Switch1/1
  Image Statistics/1 -> Switch/1
  Pixel Control Bus Selector/1 -> HDL Counter2/1  "<vEnd>"
  pixelWindow/1 -> Delay/1
  Data Type Conversion1/1 -> Divide2/1
  Subtract3/1 -> Data Type Conversion1/1
  Divide2/1 -> Delay2/1
  Switch1/1 -> Divide2/2
  Switch/1 -> Subtract3/2
  Compare To Constant1/1 -> Switch1/2, Switch/2
  Image Statistics/3 -> Terminator/1
  frameCtrl/1 -> Pixel Control Bus Selector/1
  Delay/1 -> Product/1
  Delay1/1 -> pixelOut/1
  Delay2/1 -> Product/2
  Delay3/1 -> ctrlOut/1

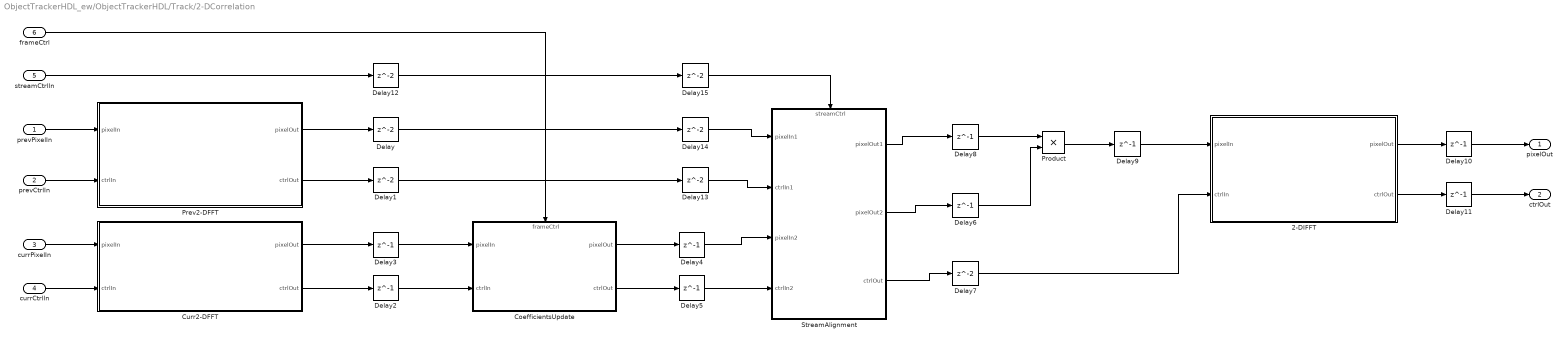
== system ObjectTrackerHDL_ew/ObjectTrackerHDL/Track/2-DCorrelation ==
  prevPixelIn : Inport
  prevCtrlIn : Inport  Port=2
  currPixelIn : Inport  Port=3
  currCtrlIn : Inport  Port=4
  streamCtrlIn : Inport  Port=5
  frameCtrl : Inport  Port=6
  2-DIFFT : Subsystem
  CoefficientsUpdate : Subsystem
      settings: PortSchema="{\"entries\":[{\"content\":{\"sides\":[{\"content\":{\"connectorIds\":[\"In1\",\"In2\"]},\"type\":\"ConnectorPlacement.EquallySpacedRectSide\",\"uuid\":\"53bd0d58-b6dc-4b0b-b458-9b3186c3348a\"},{\"content\":{\"connectorIds\":[\"Out1\",\"Out2\"],\"side\":\"RIGHT\"},\"type\":\"ConnectorPlacement.EquallySpacedRectSide\",\"uuid\":\"75a88d65-c417-47d5-912f-7fdd4f635d52\"},{\"content\":{\"connectorIds\":[\"In3\"],\"side\":\"TOP\"},\"type\":\"ConnectorPlacement.EquallySpacedRectSide\",\"uuid\":\"7478dca4-19bb-4420-a52f-60a62fa585cf\"},{\"content\":{\"side\":\"BOTTOM\"},\"type\":\"ConnectorPlacement.EquallySpacedRectSide\",\"uuid\":\"87c5ca16-ea52-46b6-b216-72fdc9c2005a\"}]},\"type\":\"ConnectorPlacement.EquallySpacedConnector\",\"uuid\":\"9c834610-d2c0-47cb-b24c-e88298881fe1\"}],\"packageUris\":[\"http://schema.mathworks.com/mf0/Connector/R2020b\"],\"version\":\"1.0\"}"
  Curr2-DFFT : Subsystem
  Delay{,1,7,12..15} (7 alike) : Delay
  Delay{2..6,8..11} (9 alike) : Delay  DelayLength=1
  Prev2-DFFT : Subsystem
  Product : Product  OutDataTypeStr=fixdt(1,24,16)
  StreamAlignment : Subsystem
      settings: PortSchema="{\"entries\":[{\"content\":{\"sides\":[{\"content\":{\"connectorIds\":[\"In1\",\"In2\",\"In3\",\"In4\"]},\"type\":\"ConnectorPlacement.EquallySpacedRectSide\",\"uuid\":\"f965da07-5f9b-4505-8661-9f286a7a9695\"},{\"content\":{\"connectorIds\":[\"Out1\",\"Out2\",\"Out3\"],\"side\":\"RIGHT\"},\"type\":\"ConnectorPlacement.EquallySpacedRectSide\",\"uuid\":\"3fb83279-f832-4878-aa73-bec98f373364\"},{\"content\":{\"connectorIds\":[\"In5\"],\"side\":\"TOP\"},\"type\":\"ConnectorPlacement.EquallySpacedRectSide\",\"uuid\":\"c47abd9b-832d-4fee-bade-9d02027f332f\"}]},\"type\":\"ConnectorPlacement.EquallySpacedConnector\",\"uuid\":\"74bc1f55-80b2-4ee4-a155-299e9ac8ba34\"}],\"packageUris\":[\"http://schema.mathworks.com/mf0/Connector/R2020b\"],\"version\":\"1.0\"}"
  pixelOut : Outport
  ctrlOut : Outport  Port=2
  wires:
  Curr2-DFFT/1(pixelOut) -> Delay3/1
  Product/1 -> Delay9/1
  prevPixelIn/1 -> Prev2-DFFT/1(pixelIn)
  StreamAlignment/1(pixelOut1) -> Delay8/1
  StreamAlignment/2(pixelOut2) -> Delay6/1
  StreamAlignment/3(ctrlOut) -> Delay7/1
  currPixelIn/1 -> Curr2-DFFT/1(pixelIn)
  prevCtrlIn/1 -> Prev2-DFFT/2(ctrlIn)
  streamCtrlIn/1 -> Delay12/1
  currCtrlIn/1 -> Curr2-DFFT/2(ctrlIn)
  2-DIFFT/1(pixelOut) -> Delay10/1
  2-DIFFT/2(ctrlOut) -> Delay11/1
  Prev2-DFFT/1(pixelOut) -> Delay/1
  Prev2-DFFT/2(ctrlOut) -> Delay1/1
  CoefficientsUpdate/1(pixelOut) -> Delay4/1
  CoefficientsUpdate/2(ctrlOut) -> Delay5/1
  Delay/1 -> Delay14/1
  Delay1/1 -> Delay13/1
  Delay2/1 -> CoefficientsUpdate/2(ctrlIn)
  Delay3/1 -> CoefficientsUpdate/1(pixelIn)
  Delay4/1 -> StreamAlignment/3(pixelIn2)
  Delay5/1 -> StreamAlignment/4(ctrlIn2)
  Delay6/1 -> Product/2
  Delay7/1 -> 2-DIFFT/2(ctrlIn)
  Delay8/1 -> Product/1
  Delay9/1 -> 2-DIFFT/1(pixelIn)
  Delay10/1 -> pixelOut/1
  Delay11/1 -> ctrlOut/1
  Curr2-DFFT/2(ctrlOut) -> Delay2/1
  Delay12/1 -> Delay15/1
  frameCtrl/1 -> CoefficientsUpdate/3(frameCtrl)
  Delay13/1 -> StreamAlignment/2(ctrlIn1)
  Delay14/1 -> StreamAlignment/1(pixelIn1)
  Delay15/1 -> StreamAlignment/5(streamCtrl)

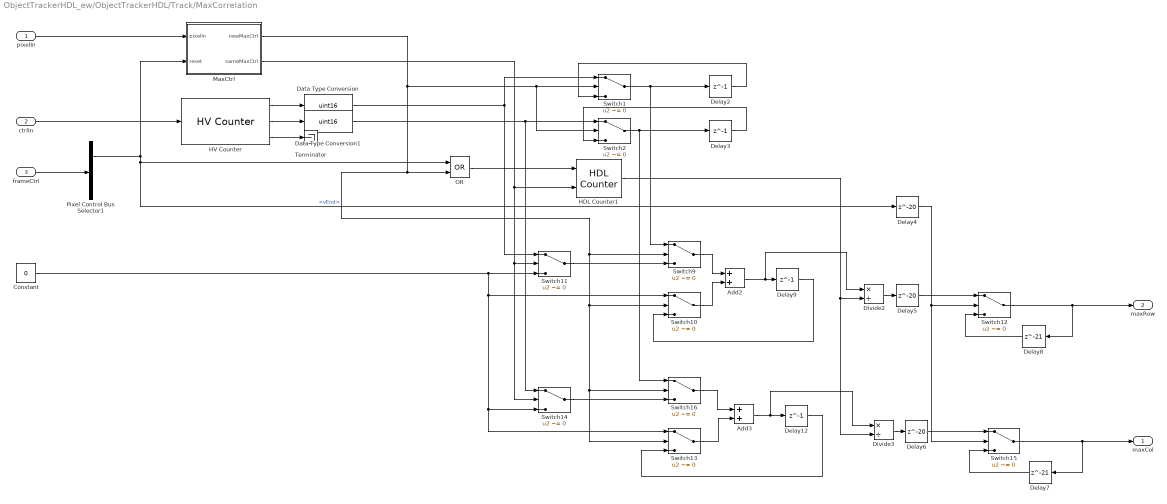
== system ObjectTrackerHDL_ew/ObjectTrackerHDL/Track/MaxCorrelation ==
  pixelIn : Inport
  ctrlIn : Inport  Port=2
  frameCtrl : Inport  Port=3
  Add2 : Sum  OutDataTypeStr=Inherit: Same as first input
  Add3 : Sum  OutDataTypeStr=Inherit: Same as first input
  Constant : Constant  Value=0  OutDataTypeStr=uint8  SampleTime=-1
  Data Type Conversion : DataTypeConversion  OutDataTypeStr=uint16  SaturateOnIntegerOverflow=off  RndMeth=Floor
  Data Type Conversion1 : DataTypeConversion  OutDataTypeStr=uint16  SaturateOnIntegerOverflow=off  RndMeth=Floor
  Delay{2..3,9,12} (4 alike) : Delay  DelayLength=1
  Delay4 : Delay  DelayLength=20
  Delay5 : Delay  DelayLength=20
  Delay6 : Delay  DelayLength=20
  Delay7 : Delay  DelayLength=21
  Delay8 : Delay  DelayLength=21
  Divide2 : Product  Inputs=*/  RndMeth=Zero  SaturateOnIntegerOverflow=on
  Divide3 : Product  Inputs=*/  RndMeth=Zero  SaturateOnIntegerOverflow=on
  HDL Counter1 : hdlsllib/Sources/HDL Counter  CountType=Free running  CountInit=1  CountStep=1  CountMax=25  CountFromType=Initial value  CountFrom=1  CountResetPort=on  CountLoadPort=off  CountEnbPort=on  CountDirPort=off  CountHitOutputPort=off  CountDataType=Unsigned  CountWordLen=16  CountFracLen=0  CountSampTime=1
  HV Counter : visionhdlutilities/HV Counter  ActivePixelsPerLine=tSize  ActiveVideoLines=tSize  SimulateUsing=Code generation
  MaxCtrl : Subsystem
  OR : Logic  Operator=OR  AllPortsSameDT=off  OutDataTypeStr=boolean
  Pixel Control Bus Selector1 : BusSelector  OutputSignals=vEnd,vStart
  Switch{1..2,9..16} (10 alike) : Switch  Criteria=u2 ~= 0  SaturateOnIntegerOverflow=off  InputSameDT=off
  Terminator : Terminator
  maxCol : Outport
  maxRow : Outport  Port=2
  wires:
  Delay9/1 -> Switch10/3
  Delay12/1 -> Switch13/3
  Switch2/1 -> Delay3/1, Switch16/1
  Switch16/1 -> Add3/1
  ctrlIn/1 -> HV Counter/1
  Data Type Conversion1/1 -> Switch14/1, Switch2/1
  Switch14/1 -> Switch16/3
  Switch9/1 -> Add2/1
  Switch1/1 -> Switch9/1, Delay2/1
  Switch13/1 -> Add3/2
  Switch11/1 -> Switch9/3
  Divide3/1 -> Delay6/1
  OR/1 -> HDL Counter1/1
  HV Counter/2 -> Data Type Conversion1/1
  Divide2/1 -> Delay5/1
  Add3/1 -> Divide3/1, Delay12/1
  Switch10/1 -> Add2/2
  Delay3/1 -> Switch2/3
  Data Type Conversion/1 -> Switch1/1, Switch11/1
  HV Counter/1 -> Data Type Conversion/1
  Delay2/1 -> Switch1/3
  HDL Counter1/1 -> Divide2/2, Divide3/2
  Add2/1 -> Divide2/1, Delay9/1
  HV Counter/3 -> Terminator/1
  Constant/1 -> Switch10/1, Switch13/1, Switch14/3, Switch11/3
  MaxCtrl/2(sameMaxCtrl) -> HDL Counter1/2, Switch11/2, Switch14/2
  MaxCtrl/1(newMaxCtrl) -> Switch13/2, Switch16/2, Switch10/2, Switch9/2, OR/2, Switch2/2, Switch1/2
  pixelIn/1 -> MaxCtrl/1(pixelIn)
  frameCtrl/1 -> Pixel Control Bus Selector1/1
  Switch12/1 -> Delay8/1, maxRow/1
  Switch15/1 -> Delay7/1, maxCol/1
  Pixel Control Bus Selector1/1 -> Delay4/1, OR/1, MaxCtrl/2(reset)  "<vEnd>"
  Delay4/1 -> Switch12/2, Switch15/2
  Delay5/1 -> Switch12/1
  Delay6/1 -> Switch15/1
  Delay7/1 -> Switch15/3
  Delay8/1 -> Switch12/3
